simulink model "gatingpulses"  (R2018a)
settings: Solver=VariableStepAuto  StartTime=0.0  StopTime=0.1  RelTol=1e-3
libraries: powerlib x13, simulink x4
settings Model: Creator=rob24  LastModifiedBy=USER

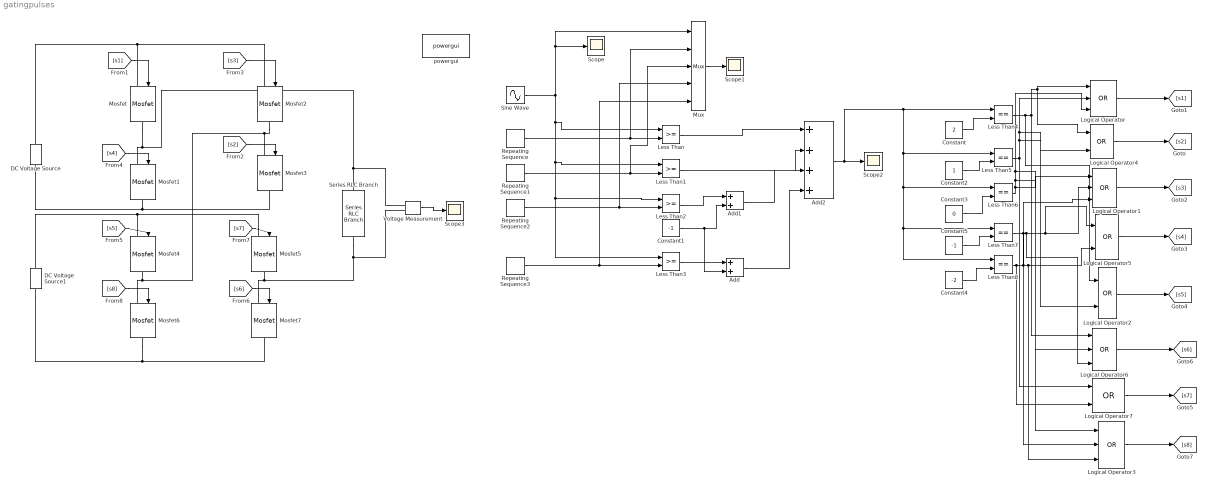
== system gatingpulses ==
  Add : Sum
  Add1 : Sum
  Add2 : Sum  Inputs=++++
  Constant : Constant  Value=2
  Constant1 : Constant  Value=-1
  Constant2 : Constant
  Constant3 : Constant  Value=0
  Constant4 : Constant  Value=-2
  Constant5 : Constant  Value=-1
  DC Voltage Source : powerlib/Electrical Sources/DC Voltage Source  Amplitude=100  Measurements=None
  DC Voltage Source1 : powerlib/Electrical Sources/DC Voltage Source  Amplitude=100  Measurements=None
  Less Than{,1..3} (4 alike) : RelationalOperator  OutDataTypeStr=boolean  RndMeth=Simplest
  Less Than{4..8} (5 alike) : RelationalOperator  Operator===  OutDataTypeStr=boolean  RndMeth=Simplest
  Logical Operator{,1,3,6} (4 alike) : Logic  Operator=OR  Inputs=3  AllPortsSameDT=off  OutDataTypeStr=boolean
  Logical Operator{2,4..5,7} (4 alike) : Logic  Operator=OR  AllPortsSameDT=off  OutDataTypeStr=boolean
  Mosfet{,1..7} (8 alike) : powerlib/Power Electronics/Mosfet  Ron=0.1  Lon=0  Rd=0.01  Vfd=0  IC=0  Rs=1e5  Cs=inf  Measurements=off
  Mux : Mux  Inputs=5
  Repeating Sequence : simulink/Sources/Repeating Sequence  rep_seq_t=[0 1/2000 1/1000]  rep_seq_y=[1 2 1]
  Repeating Sequence1 : simulink/Sources/Repeating Sequence  rep_seq_t=[0 1/2000 1/1000]  rep_seq_y=[0 1 0]
  Repeating Sequence2 : simulink/Sources/Repeating Sequence  rep_seq_t=[0 1/2000 1/1000]  rep_seq_y=[0 -1 0]
  Repeating Sequence3 : simulink/Sources/Repeating Sequence  rep_seq_t=[0 1/2000 1/1000]  rep_seq_y=[-1 -2 1]
  Scope{,1..3} (4 alike) : Scope
  Series RLC Branch : powerlib/Elements/Series RLC Branch  LConnTagsString=__new0  RConnTagsString=__new0  BranchType=RL  Resistance=25  Inductance=1e-3  SetiL0=off  InitialCurrent=0  Capacitance=1e-6  Setx0=off  InitialVoltage=0  Measurements=None
  Sine Wave : Sin  Amplitude=(0.85*2)  Frequency=2*pi*50  SampleTime=1e-6
  Voltage Measurement : powerlib/Measurements/Voltage Measurement  PhasorSimulation=off  OutputType=Complex  PSBequivalent=0
  powergui : powerlib/powergui  Priority=1  SimulationMode=Continuous  SampleTime=50e-6  frequency=60  Iterations=50  frequencyindice=0  Pbase=100e6  ErrMax=1e-4  UnitsV=kV  UnitsW=MW  buscounter=0  FunctionMessages=off  echomessages=off  EnableUseOfTLC=off  CurrentSourceSwitches=off  DisableSnubberDevices=off  DisableRonSwitches=off  DisableVfSwitches=off  DisplayEquations=off  SolverType=Tustin/Backward Euler (TBE)  Interpol=off  ExternalGateDelay=off  methode=off  Ts=100  x0status=blocks  SPID=on  SwTol=0  HookPort=off  RestoreLinks=warning  ResistiveCurrentMeasurement=off  Frange=[0:2:500]  Ylog=off  Xlog=on  ShowGrid=off  save=off  variable=ZData  structure=0  ZoomFFT=off  StartTime=0.0  cycles=1  DisplayStyle=1  fundamental=60  FreqAxis=off  MaxFrequency=1000  frequencyindicesteady=1  RmsSteady=1  display=off
  wires:
  Repeating Sequence/1 -> Mux/2, Less Than/2
  Repeating Sequence1/1 -> Mux/3, Less Than1/2
  Repeating Sequence2/1 -> Mux/4, Less Than2/2
  Repeating Sequence3/1 -> Mux/5, Less Than3/2
  Sine Wave/1 -> Less Than/1, Less Than1/1, Less Than2/1, Less Than3/1, Scope/1, Mux/1
  Mux/1 -> Scope1/1
  Less Than2/1 -> Add1/1
  Constant1/1 -> Add/2, Add1/2
  Less Than3/1 -> Add/1
  Less Than/1 -> Add2/1
  Less Than1/1 -> Add2/2
  Add1/1 -> Add2/3
  Add/1 -> Add2/4
  Constant/1 -> Less Than4/2
  Constant4/1 -> Less Than8/2
  Constant5/1 -> Less Than7/2
  Constant3/1 -> Less Than6/2
  Constant2/1 -> Less Than5/2
  Add2/1 -> Less Than5/1, Less Than6/1, Less Than7/1, Less Than8/1, Less Than4/1, Scope2/1
  Logical Operator/1 -> [s1]
  Logical Operator4/1 -> [s2]
  Logical Operator1/1 -> [s3]
  Logical Operator5/1 -> [s4]
  Logical Operator2/1 -> [s5]
  Logical Operator6/1 -> [s6]
  Logical Operator7/1 -> [s7]
  Logical Operator3/1 -> [s8]
  Less Than4/1 -> Logical Operator2/1, Logical Operator6/1, Logical Operator4/1, Logical Operator/1
  Less Than5/1 -> Logical Operator7/1, Logical Operator2/2, Logical Operator4/2, Logical Operator/2
  Less Than6/1 -> Logical Operator1/1, Logical Operator3/1, Logical Operator6/2, Logical Operator/3
  Less Than7/1 -> Logical Operator1/2, Logical Operator5/1, Logical Operator6/3, Logical Operator3/2
  Less Than8/1 -> Logical Operator7/2, Logical Operator1/3, Logical Operator3/3, Logical Operator5/2
  [s3] -> Mosfet2/1
  [s1] -> Mosfet/1
  [s2] -> Mosfet3/1
  [s4] -> Mosfet1/1
  [s7] -> Mosfet5/1
  [s5] -> Mosfet4/1
  [s6] -> Mosfet7/1
  [s8] -> Mosfet6/1
  Voltage Measurement/1 -> Scope3/1
  connections:
  Mosfet5/LConn1 -- Mosfet4/LConn1 -- DC Voltage Source1/RConn1
  DC Voltage Source1/LConn1 -- Mosfet6/RConn1 -- Mosfet7/RConn1
  Mosfet5/RConn1 -- Voltage Measurement/LConn2 -- Series RLC Branch/RConn1 -- Mosfet7/LConn1
  DC Voltage Source/LConn1 -- Mosfet1/RConn1 -- Mosfet3/RConn1
  Mosfet2/RConn1 -- Mosfet4/RConn1 -- Mosfet6/LConn1 -- Mosfet3/LConn1
  Mosfet/RConn1 -- Voltage Measurement/LConn1 -- Series RLC Branch/LConn1 -- Mosfet1/LConn1
  DC Voltage Source/RConn1 -- Mosfet/LConn1 -- Mosfet2/LConn1
